simulink model "simulare_regulator_etapa1"  (R2020a)
settings: Solver=VariableStepAuto  StartTime=0.0  StopTime=500  RelTol=1e-3
settings Model: Creator=user  LastModifiedBy=user

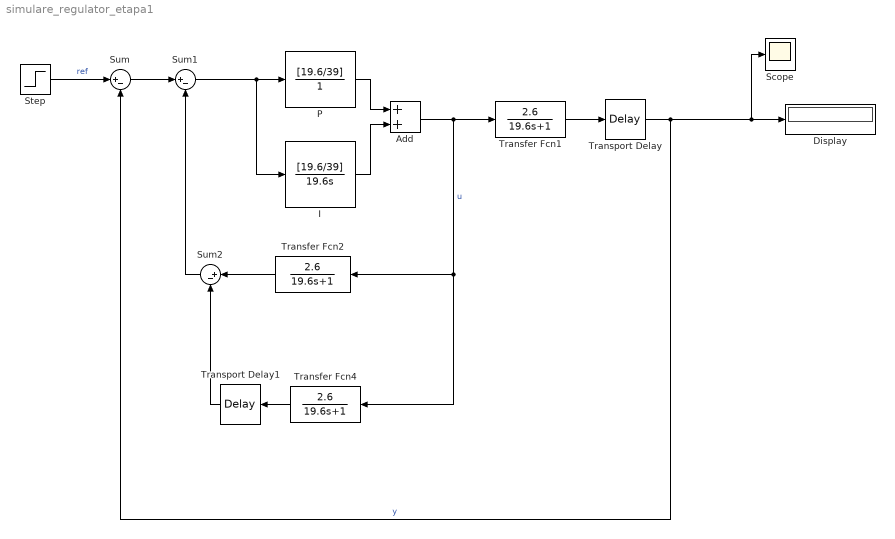
== system simulare_regulator_etapa1 ==
  Add : Sum
  Display : Display
  I : TransferFcn  Numerator=[19.6/39]  Denominator=[19.6 0]
  P : TransferFcn  Numerator=[19.6/39]  Denominator=[0 1]
  Scope : Scope
  Step : Step  SampleTime=0
  Sum : Sum  Inputs=|+-
  Sum1 : Sum  Inputs=|+-
  Sum2 : Sum  Inputs=|+-
  Transfer Fcn1 : TransferFcn  Numerator=[2.6]  Denominator=[19.6 1]
  Transfer Fcn2 : TransferFcn  Numerator=[2.6]  Denominator=[19.6 1]
  Transfer Fcn4 : TransferFcn  Numerator=[2.6]  Denominator=[19.6 1]
  Transport Delay : TransportDelay  DelayTime=5
  Transport Delay1 : TransportDelay  DelayTime=5
  wires:
  Step/1 -> Sum/1  "ref"
  Sum/1 -> Sum1/1
  Sum1/1 -> I/1, P/1
  P/1 -> Add/1
  I/1 -> Add/2
  Add/1 -> Transfer Fcn4/1, Transfer Fcn2/1, Transfer Fcn1/1  "u"
  Transfer Fcn1/1 -> Transport Delay/1
  Transport Delay/1 -> Scope/1, Display/1, Sum/2  "y"
  Transfer Fcn4/1 -> Transport Delay1/1
  Transfer Fcn2/1 -> Sum2/1
  Transport Delay1/1 -> Sum2/2
  Sum2/1 -> Sum1/2
